simulink model "blank_canvas_curr_MR"  (R2025b)
settings: Solver=FixedStepAuto  StartTime=0.0  StopTime=2  FixedStep=Ts  RelTol=1e-3
undefined symbols (not defined in the file or in its folder): Ts
settings Model: Creator=gdudgeon  LastModifiedBy=gdudgeon
settings DataIOCC: SaveOutput=off  SignalLogging=off  DSMLogging=off  SaveTime=off  ReturnWorkspaceOutputs=off
settings RTWCC: GPUComputeCapability=3.5

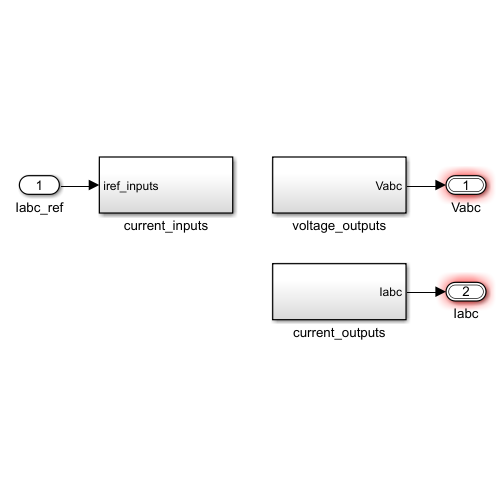
[thumbnail: Simulink's stored preview of the top-level diagram]
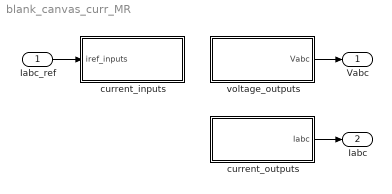
== system blank_canvas_curr_MR ==
  Iabc_ref : Inport
  current_inputs : Subsystem
  current_outputs : Subsystem
  voltage_outputs : Subsystem
  Vabc : Outport  OutDataTypeStr=Bus: slBus1  SampleTime=Ts
  Iabc : Outport  Port=2  OutDataTypeStr=Bus: slBus2  SampleTime=Ts
  wires:
  voltage_outputs/1(Vabc) -> Vabc/1
  current_outputs/1(Iabc) -> Iabc/1
  Iabc_ref/1 -> current_inputs/1(iref_inputs)

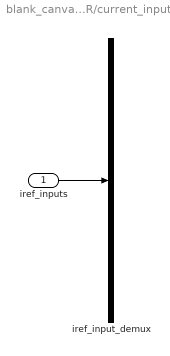
== system blank_canvas_curr_MR/current_inputs ==
  iref_inputs : Inport
  iref_input_demux : Demux  Outputs=2
  wires:
  iref_inputs/1 -> iref_input_demux/1

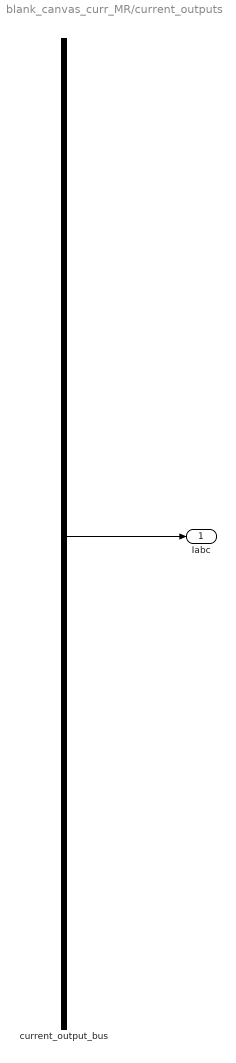
== system blank_canvas_curr_MR/current_outputs ==
  current_output_bus : BusCreator  Inputs=2
  Iabc : Outport  OutDataTypeStr=Bus: slBus2  SampleTime=Ts  VectorParamsAs1DForOutWhenUnconnected=off
  wires:
  current_output_bus/1 -> Iabc/1

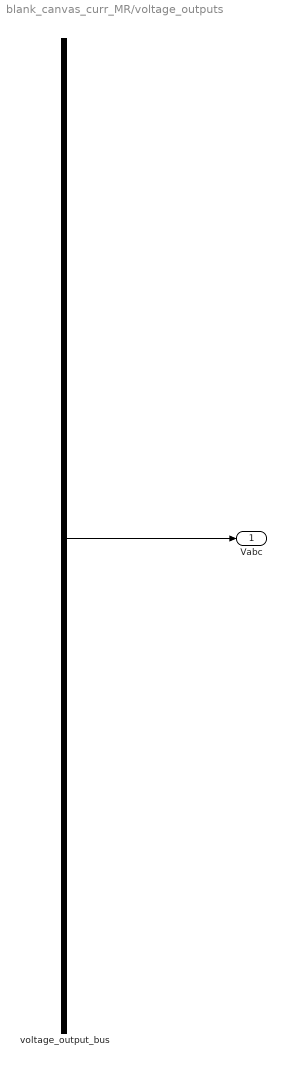
== system blank_canvas_curr_MR/voltage_outputs ==
  voltage_output_bus : BusCreator  Inputs=2
  Vabc : Outport  OutDataTypeStr=Bus: slBus1  SampleTime=Ts  VectorParamsAs1DForOutWhenUnconnected=off
  wires:
  voltage_output_bus/1 -> Vabc/1
